simulink model "ExRobotAndEnvironmentController"  (Simulink 8.7)
settings: Solver=ode45  StartTime=0.0  StopTime=1000  FixedStep=.01  RelTol=1e-3
values from neighbouring files (symbols this model uses):
  distanceMin = 20    [InitRobotAndEnvironment.m]
  INITIAL_ROBOT_POS_THETA = 1.5    [InitRobotAndEnvironment.m]
  INITIAL_ROBOT_POS_X = 0    [InitRobotAndEnvironment.m]
  INITIAL_ROBOT_POS_Y = 0    [InitRobotAndEnvironment.m]
  INTER_WHEEL_DISTANCE = 0.12    [InitRobotAndEnvironment.m]
  ki_teta = omega*omega/alpha    (= 0.2)    [InitRobotAndEnvironment.m]
  kp_teta = 2*ksi*omega/alpha    (= 0.4)    [InitRobotAndEnvironment.m]
  MAX_SPEED = .5    (= 0.5)    [InitRobotAndEnvironment.m]
  ts = SENSOR_SAMPLING_TIME    (= 0.001)    [InitRobotAndEnvironment.m]
  ts_anim = ANIMATION_SAMPLING_TIME    (= 0.01)    [InitRobotAndEnvironment.m]
undefined symbols (not defined in the file or in its folder): Env, Robot, RobotInit
libraries: simulink x3
settings Model: Creator=alex  LastModifiedBy=bonnajul
settings OptimizationCC: ExpressionDepthLimit=2147483647
settings DebuggingCC: FcnCallInpInsideContextMsg=UseLocalSettings  StateNameClashWarn=warning
settings SFSimCC: SimParseCustomCode=off
settings GRTTargetCC: CombineOutputUpdateFcns=off  GRTInterface=on

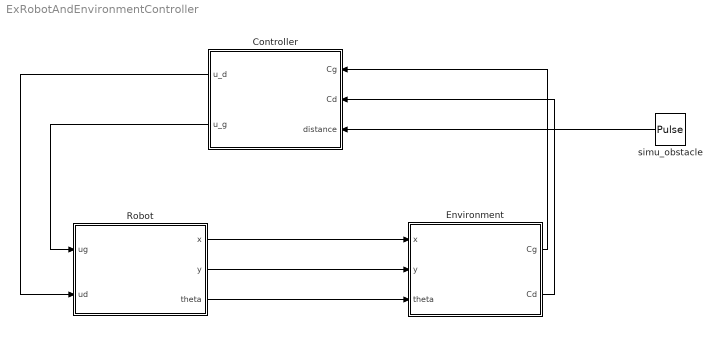
== system ExRobotAndEnvironmentController ==
  Controller : Subsystem
  Environment : Subsystem
  Robot : Subsystem
  "simu_obstacle " : DiscretePulseGenerator  PulseType=Time based  Amplitude=30  Period=3  PulseWidth=80
  wires:
  Controller/1(u_d) -> Robot/2(ud)
  Controller/2(u_g) -> Robot/1(ug)
  Robot/1(x) -> Environment/1(x)
  Robot/3(theta) -> Environment/3(theta)
  Robot/2(y) -> Environment/2(y)
  Environment/2(Cd) -> Controller/2(Cd)
  Environment/1(Cg) -> Controller/1(Cg)
  "simu_obstacle "/1 -> Controller/3(distance)

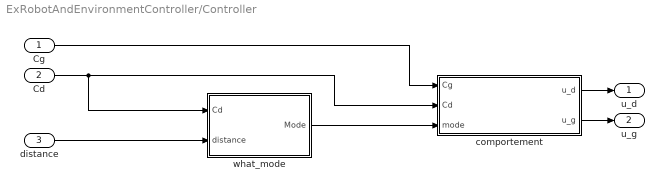
== system ExRobotAndEnvironmentController/Controller ==
  Cg : Inport
  Cd : Inport  Port=2
  distance : Inport  Port=3
  comportement : Subsystem
  what_mode : Subsystem
  u_d : Outport
  u_g : Outport  Port=2
  wires:
  Cd/1 -> what_mode/1(Cd), comportement/2(Cd)
  distance/1 -> what_mode/2(distance)
  Cg/1 -> comportement/1(Cg)
  what_mode/1(Mode) -> comportement/3(mode)
  comportement/1(u_d) -> u_d/1
  comportement/2(u_g) -> u_g/1

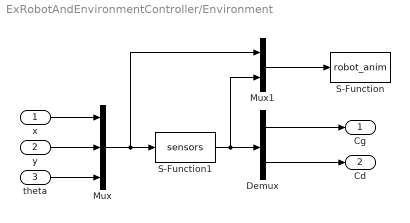
== system ExRobotAndEnvironmentController/Environment ==
  x : Inport
  y : Inport  Port=2
  theta : Inport  Port=3
  Demux : Demux  Outputs=2
  Mux : Mux  Inputs=3
  Mux1 : Mux  Inputs=2
  S-Function : S-Function  FunctionName=robot_anim  Parameters=ts_anim,Env,Robot,RobotInit  SFunctionDeploymentMode=off  EnableBusSupport=off
  S-Function1 : S-Function  FunctionName=sensors  Parameters=ts,Env,Robot  SFunctionDeploymentMode=off  EnableBusSupport=off
  Cg : Outport
  Cd : Outport  Port=2
  wires:
  x/1 -> Mux/1
  y/1 -> Mux/2
  theta/1 -> Mux/3
  Mux/1 -> S-Function1/1, Mux1/1
  S-Function1/1 -> Mux1/2, Demux/1
  Mux1/1 -> S-Function/1
  Demux/1 -> Cg/1
  Demux/2 -> Cd/1

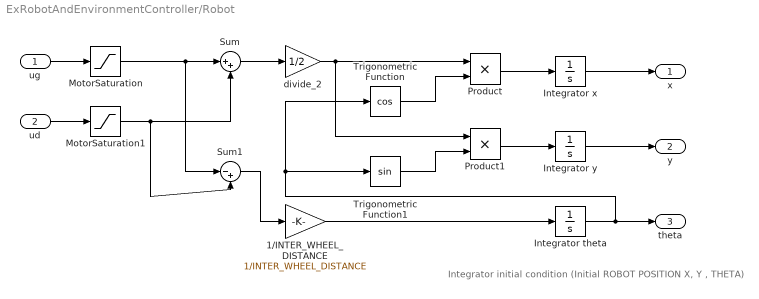
== system ExRobotAndEnvironmentController/Robot ==
  note: Integrator initial condition (Initial ROBOT POSITION X, Y , THETA)
  ug : Inport
  ud : Inport  Port=2
  1/INTER_WHEEL_DISTANCE : Gain  Gain=1/INTER_WHEEL_DISTANCE
  Integrator theta : Integrator  InitialCondition=INITIAL_ROBOT_POS_THETA
  Integrator x : Integrator  InitialCondition=INITIAL_ROBOT_POS_X
  Integrator y : Integrator  InitialCondition=INITIAL_ROBOT_POS_Y
  MotorSaturation : Saturate  UpperLimit=MAX_SPEED  LowerLimit=-MAX_SPEED
  MotorSaturation1 : Saturate  UpperLimit=MAX_SPEED  LowerLimit=-MAX_SPEED
  Product : Product  RndMeth=Zero
  Product1 : Product  RndMeth=Zero
  Sum : Sum  Inputs=|++
  Sum1 : Sum  Inputs=|-+
  Trigonometric Function : Trigonometry  Operator=cos
  Trigonometric Function1 : Trigonometry
  divide_2 : Gain  Gain=1/2
  x : Outport
  y : Outport  Port=2
  theta : Outport  Port=3
  wires:
  ug/1 -> MotorSaturation/1
  Integrator x/1 -> x/1
  Integrator y/1 -> y/1
  Integrator theta/1 -> Trigonometric Function/1, Trigonometric Function1/1, theta/1
  Sum/1 -> divide_2/1
  divide_2/1 -> Product1/1, Product/1
  Trigonometric Function/1 -> Product/2
  Trigonometric Function1/1 -> Product1/2
  Product/1 -> Integrator x/1
  Product1/1 -> Integrator y/1
  Sum1/1 -> 1/INTER_WHEEL_DISTANCE/1
  1/INTER_WHEEL_DISTANCE/1 -> Integrator theta/1
  ud/1 -> MotorSaturation1/1
  MotorSaturation1/1 -> Sum/2, Sum1/2
  MotorSaturation/1 -> Sum/1, Sum1/1

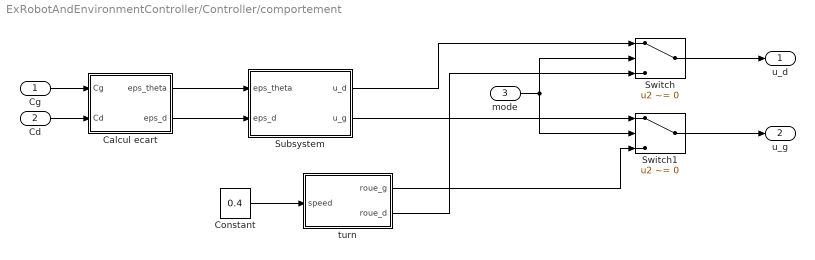
== system ExRobotAndEnvironmentController/Controller/comportement ==
  Cg : Inport
  Cd : Inport  Port=2
  mode : Inport  Port=3  OutDataTypeStr=boolean
  Calcul ecart : Subsystem
  Constant : Constant  Value=0.4
  Subsystem : Subsystem
  Switch : Switch  Criteria=u2 ~= 0
  Switch1 : Switch  Criteria=u2 ~= 0
  turn : Subsystem
  u_d : Outport
  u_g : Outport  Port=2
  wires:
  Cd/1 -> Calcul ecart/2(Cd)
  Constant/1 -> turn/1(speed)
  Calcul ecart/2(eps_d) -> Subsystem/2(eps_d)
  Cg/1 -> Calcul ecart/1(Cg)
  Calcul ecart/1(eps_theta) -> Subsystem/1(eps_theta)
  Switch1/1 -> u_g/1
  Switch/1 -> u_d/1
  Subsystem/1(u_d) -> Switch/1
  Subsystem/2(u_g) -> Switch1/1
  turn/1(roue_g) -> Switch1/3
  turn/2(roue_d) -> Switch/3
  mode/1 -> Switch1/2, Switch/2

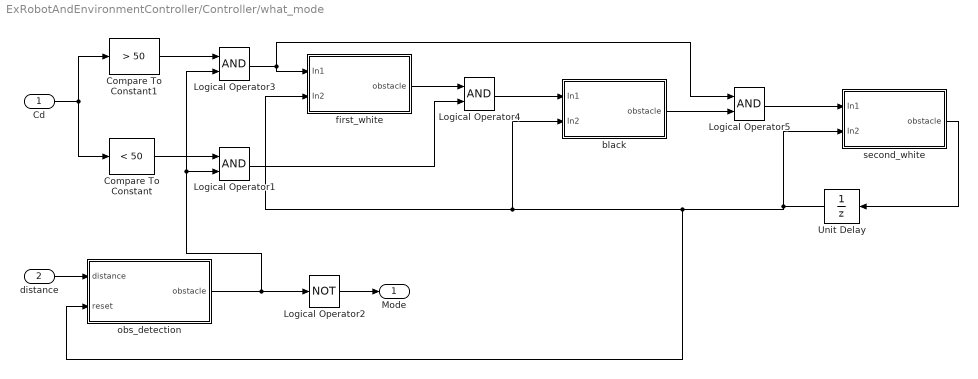
== system ExRobotAndEnvironmentController/Controller/what_mode ==
  Cd : Inport  OutDataTypeStr=double
  distance : Inport  Port=2  OutDataTypeStr=double
  Compare To Constant : simulink/Logic and Bit Operations/Compare To Constant  relop=<  const=50  OutDataTypeStr=boolean
  Compare To Constant1 : simulink/Logic and Bit Operations/Compare To Constant  relop=>  const=50  OutDataTypeStr=boolean
  Logical Operator{1,3..5} (4 alike) : Logic  AllPortsSameDT=off  OutDataTypeStr=boolean
  Logical Operator2 : Logic  Operator=NOT  AllPortsSameDT=off  OutDataTypeStr=boolean
  Unit Delay : UnitDelay  SampleTime=-1
  black : Subsystem
  first_white : Subsystem
  "obs_detection " : Subsystem
  second_white : Subsystem
  Mode : Outport
  wires:
  distance/1 -> "obs_detection "/1(distance)
  "obs_detection "/1(obstacle) -> Logical Operator2/1, Logical Operator3/2, Logical Operator1/2
  Cd/1 -> Compare To Constant/1, Compare To Constant1/1
  Compare To Constant/1 -> Logical Operator1/1
  Logical Operator2/1 -> Mode/1
  Compare To Constant1/1 -> Logical Operator3/1
  Logical Operator3/1 -> first_white/1(In1), Logical Operator5/1
  first_white/1(obstacle) -> Logical Operator4/1
  Logical Operator1/1 -> Logical Operator4/2
  Logical Operator4/1 -> black/1(In1)
  black/1(obstacle) -> Logical Operator5/2
  Logical Operator5/1 -> second_white/1(In1)
  second_white/1(obstacle) -> Unit Delay/1
  Unit Delay/1 -> "obs_detection "/2(reset), first_white/2(In2), black/2(In2), second_white/2(In2)

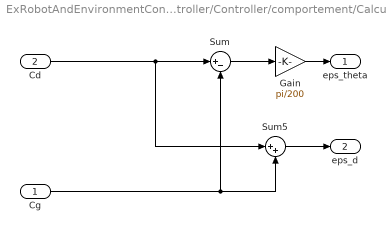
== system ExRobotAndEnvironmentController/Controller/comportement/Calcul ecart ==
  Cg : Inport
  Cd : Inport  Port=2
  Gain : Gain  Gain=pi/200
  Sum : Sum  Inputs=|+-
  Sum5 : Sum  Inputs=|++
  eps_theta : Outport
  eps_d : Outport  Port=2
  wires:
  Sum/1 -> Gain/1
  Cd/1 -> Sum/1, Sum5/1
  Cg/1 -> Sum/2, Sum5/2
  Gain/1 -> eps_theta/1
  Sum5/1 -> eps_d/1

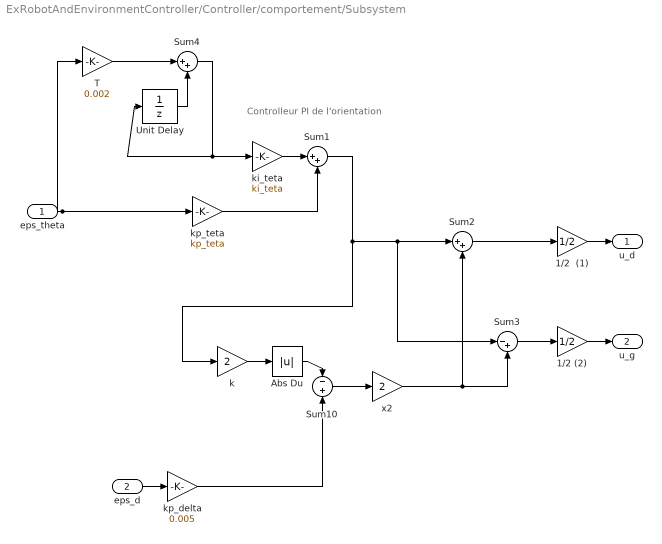
== system ExRobotAndEnvironmentController/Controller/comportement/Subsystem ==
  note: Controlleur PI de l'orientation
  eps_theta : Inport
  eps_d : Inport  Port=2
  1/2  (1) : Gain  Gain=1/2  SaturateOnIntegerOverflow=on  OutDataTypeStr=Inherit: Same as input  ParamDataTypeStr=Inherit: Same as input
  1/2 (2) : Gain  Gain=1/2  SaturateOnIntegerOverflow=on  OutDataTypeStr=Inherit: Same as input  ParamDataTypeStr=Inherit: Same as input
  Abs Du : Abs  SaturateOnIntegerOverflow=on
  Sum1 : Sum  Inputs=|++  SaturateOnIntegerOverflow=on
  Sum10 : Sum  Inputs=-+  SaturateOnIntegerOverflow=on
  Sum2 : Sum  Inputs=|++  SaturateOnIntegerOverflow=on
  Sum3 : Sum  Inputs=|-+  SaturateOnIntegerOverflow=on
  Sum4 : Sum  Inputs=|++
  T : Gain  Gain=0.002
  Unit Delay : UnitDelay  SampleTime=-1
  k : Gain  Gain=2  SaturateOnIntegerOverflow=on  OutDataTypeStr=Inherit: Same as input  ParamDataTypeStr=Inherit: Same as input
  ki_teta : Gain  Gain=ki_teta  SaturateOnIntegerOverflow=on  OutDataTypeStr=Inherit: Same as input  ParamDataTypeStr=Inherit: Same as input
  kp_delta : Gain  Gain=0.005
  kp_teta : Gain  Gain=kp_teta  SaturateOnIntegerOverflow=on  OutDataTypeStr=Inherit: Same as input  ParamDataTypeStr=Inherit: Same as input
  x2 : Gain  Gain=2  SaturateOnIntegerOverflow=on  OutDataTypeStr=Inherit: Same as input  ParamDataTypeStr=Inherit: Same as input
  u_d : Outport
  u_g : Outport  Port=2
  wires:
  ki_teta/1 -> Sum1/1
  kp_teta/1 -> Sum1/2
  Sum2/1 -> 1/2  (1)/1
  Sum3/1 -> 1/2 (2)/1
  k/1 -> Abs Du/1
  kp_delta/1 -> Sum10/2
  eps_theta/1 -> kp_teta/1, T/1
  Abs Du/1 -> Sum10/1
  x2/1 -> Sum2/2, Sum3/2
  Sum10/1 -> x2/1
  Sum1/1 -> k/1, Sum2/1, Sum3/1
  T/1 -> Sum4/1
  Sum4/1 -> ki_teta/1, Unit Delay/1
  Unit Delay/1 -> Sum4/2
  1/2  (1)/1 -> u_d/1
  1/2 (2)/1 -> u_g/1
  eps_d/1 -> kp_delta/1

== system ExRobotAndEnvironmentController/Controller/comportement/turn ==
  speed : Inport
  Gain : Gain  Gain=-1
  roue_g : Outport
  roue_d : Outport  Port=2
  wires:
  Gain/1 -> roue_d/1
  speed/1 -> Gain/1, roue_g/1

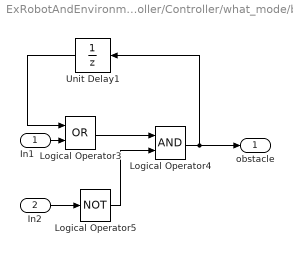
== system ExRobotAndEnvironmentController/Controller/what_mode/black ==
  In1 : Inport
  In2 : Inport  Port=2
  Logical Operator3 : Logic  Operator=OR  AllPortsSameDT=off  OutDataTypeStr=boolean
  Logical Operator4 : Logic  AllPortsSameDT=off  OutDataTypeStr=boolean
  Logical Operator5 : Logic  Operator=NOT  AllPortsSameDT=off  OutDataTypeStr=boolean
  Unit Delay1 : UnitDelay  SampleTime=-1
  obstacle : Outport
  wires:
  Logical Operator3/1 -> Logical Operator4/1
  Unit Delay1/1 -> Logical Operator3/1
  Logical Operator4/1 -> obstacle/1, Unit Delay1/1
  In1/1 -> Logical Operator3/2
  In2/1 -> Logical Operator5/1
  Logical Operator5/1 -> Logical Operator4/2

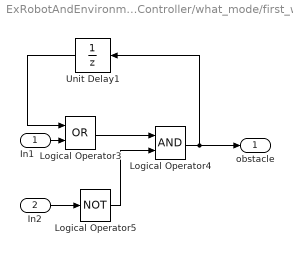
== system ExRobotAndEnvironmentController/Controller/what_mode/first_white ==
  In1 : Inport
  In2 : Inport  Port=2
  Logical Operator3 : Logic  Operator=OR  AllPortsSameDT=off  OutDataTypeStr=boolean
  Logical Operator4 : Logic  AllPortsSameDT=off  OutDataTypeStr=boolean
  Logical Operator5 : Logic  Operator=NOT  AllPortsSameDT=off  OutDataTypeStr=boolean
  Unit Delay1 : UnitDelay  SampleTime=-1
  obstacle : Outport
  wires:
  Logical Operator3/1 -> Logical Operator4/1
  Unit Delay1/1 -> Logical Operator3/1
  Logical Operator4/1 -> obstacle/1, Unit Delay1/1
  In1/1 -> Logical Operator3/2
  In2/1 -> Logical Operator5/1
  Logical Operator5/1 -> Logical Operator4/2

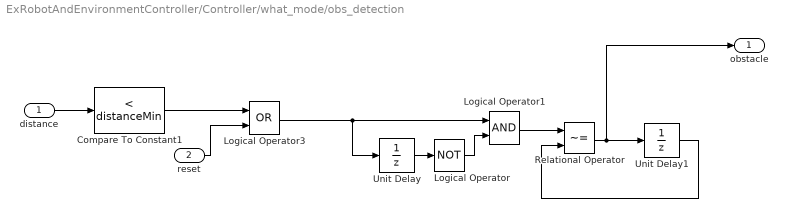
== system ExRobotAndEnvironmentController/Controller/what_mode/obs_detection  ==
  distance : Inport
  reset : Inport  Port=2
  Compare To Constant1 : simulink/Logic and Bit Operations/Compare To Constant  relop=<  const=distanceMin  OutDataTypeStr=boolean
  Logical Operator : Logic  Operator=NOT  AllPortsSameDT=off  OutDataTypeStr=boolean
  Logical Operator1 : Logic  AllPortsSameDT=off  OutDataTypeStr=boolean
  Logical Operator3 : Logic  Operator=OR  AllPortsSameDT=off  OutDataTypeStr=boolean
  Relational Operator : RelationalOperator  Operator=~=  OutDataTypeStr=boolean
  Unit Delay : UnitDelay  SampleTime=-1
  Unit Delay1 : UnitDelay  SampleTime=-1
  obstacle : Outport
  wires:
  Unit Delay/1 -> Logical Operator/1
  Unit Delay1/1 -> Relational Operator/2
  Logical Operator1/1 -> Relational Operator/1
  Logical Operator/1 -> Logical Operator1/2
  Relational Operator/1 -> obstacle/1, Unit Delay1/1
  Logical Operator3/1 -> Logical Operator1/1, Unit Delay/1
  reset/1 -> Logical Operator3/2
  distance/1 -> Compare To Constant1/1
  Compare To Constant1/1 -> Logical Operator3/1

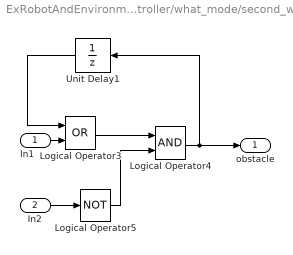
== system ExRobotAndEnvironmentController/Controller/what_mode/second_white ==
  In1 : Inport
  In2 : Inport  Port=2
  Logical Operator3 : Logic  Operator=OR  AllPortsSameDT=off  OutDataTypeStr=boolean
  Logical Operator4 : Logic  AllPortsSameDT=off  OutDataTypeStr=boolean
  Logical Operator5 : Logic  Operator=NOT  AllPortsSameDT=off  OutDataTypeStr=boolean
  Unit Delay1 : UnitDelay  SampleTime=-1
  obstacle : Outport
  wires:
  Logical Operator3/1 -> Logical Operator4/1
  Unit Delay1/1 -> Logical Operator3/1
  Logical Operator4/1 -> obstacle/1, Unit Delay1/1
  In1/1 -> Logical Operator3/2
  In2/1 -> Logical Operator5/1
  Logical Operator5/1 -> Logical Operator4/2
